simulink model "PEMFC20220411"  (R2021a)
settings: Solver=VariableStepAuto  StartTime=0.0  StopTime=3500  RelTol=1e-3
settings Model: Creator=workstation  LastModifiedBy=workstation

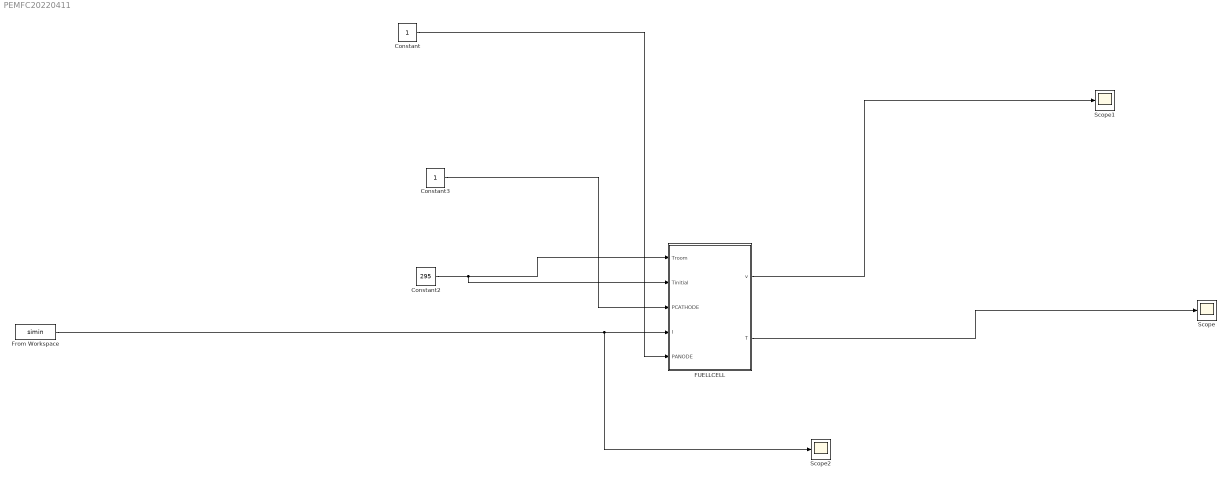
== system PEMFC20220411 ==
  Constant : Constant
  Constant2 : Constant  Value=295
  Constant3 : Constant
  FUELLCELL : Subsystem
  From Workspace : FromWorkspace  VariableName=simin
  Scope : Scope
  Scope1 : Scope
  Scope2 : Scope
  wires:
  Constant2/1 -> FUELLCELL/2(Tinitial), FUELLCELL/1(Troom)
  Constant3/1 -> FUELLCELL/3(PCATHODE)
  From Workspace/1 -> Scope2/1, FUELLCELL/4(I)
  Constant/1 -> FUELLCELL/5(PANODE)
  FUELLCELL/1(v) -> Scope1/1
  FUELLCELL/2(T) -> Scope/1

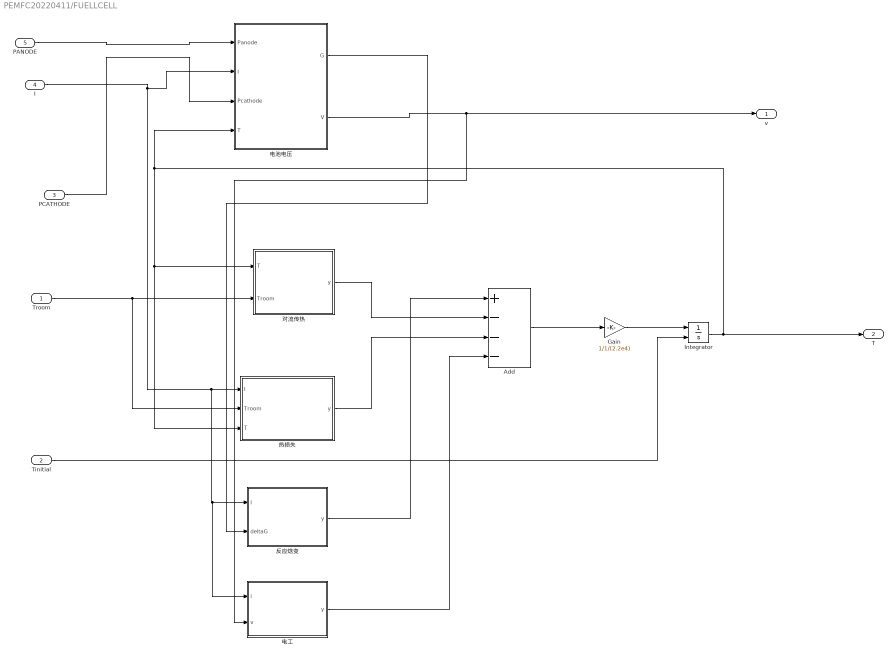
== system PEMFC20220411/FUELLCELL ==
  Troom : Inport
  Tinitial : Inport  Port=2
  PCATHODE : Inport  Port=3
  I : Inport  Port=4
  PANODE : Inport  Port=5
  Add : Sum  Inputs=+---
  Gain : Gain  Gain=1/1/(2.2e4)
  Integrator : Integrator  InitialConditionSource=external
  反应焓变 : MATLAB Function  TreatAsAtomicUnit=on
  对流传热 : MATLAB Function  TreatAsAtomicUnit=on
  热损失 : MATLAB Function  TreatAsAtomicUnit=on
  电工 : MATLAB Function  TreatAsAtomicUnit=on
  电池电压 : Subsystem
  v : Outport
  T : Outport  Port=2
  wires:
  电池电压/2(V) -> v/1, 电工/2(v)
  Integrator/1 -> T/1, 电池电压/4(T), 热损失/3(T), 对流传热/1(T)
  对流传热/1(y) -> Add/2
  Troom/1 -> 热损失/2(Troom), 对流传热/2(Troom)
  Gain/1 -> Integrator/1
  Tinitial/1 -> Integrator/2
  PANODE/1 -> 电池电压/1(Panode)
  热损失/1(y) -> Add/3
  I/1 -> 电工/1(i), 反应焓变/1(I), 热损失/1(I), 电池电压/2(I)
  电池电压/1(G) -> 反应焓变/2(deltaG)
  反应焓变/1(y) -> Add/1
  Add/1 -> Gain/1
  PCATHODE/1 -> 电池电压/3(Pcathode)
  电工/1(y) -> Add/4

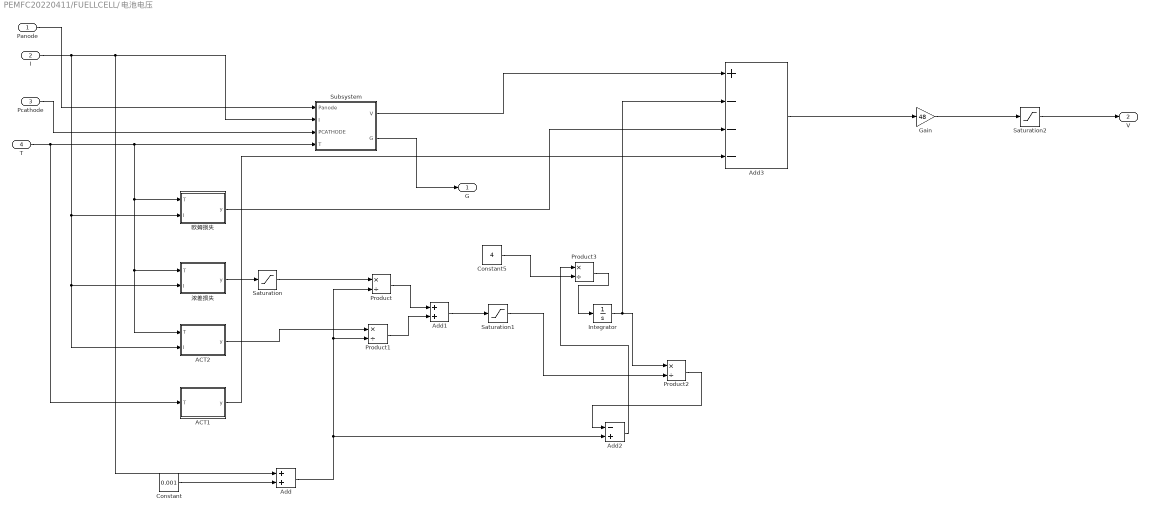
== system PEMFC20220411/FUELLCELL/电池电压 ==
  Panode : Inport
  I : Inport  Port=2
  Pcathode : Inport  Port=3
  T : Inport  Port=4
  ACT1 : MATLAB Function  TreatAsAtomicUnit=on
  ACT2 : MATLAB Function  TreatAsAtomicUnit=on
  Add : Sum
  Add1 : Sum
  Add2 : Sum  Inputs=-+
  Add3 : Sum  Inputs=+---
  Constant : Constant  Value=0.001
  Constant5 : Constant  Value=4
  Gain : Gain  Gain=48
  Integrator : Integrator
  Product{,1..3} (4 alike) : Product  Inputs=*/
  Saturation : Saturate  UpperLimit=1  LowerLimit=0
  Saturation1 : Saturate  UpperLimit=10  LowerLimit=0.00001
  Saturation2 : Saturate  UpperLimit=58  LowerLimit=0
  Subsystem : Subsystem
  欧姆损失 : MATLAB Function  TreatAsAtomicUnit=on
  浓差损失 : MATLAB Function  TreatAsAtomicUnit=on
  G : Outport
  V : Outport  Port=2
  wires:
  Add2/1 -> Product3/1
  Pcathode/1 -> Subsystem/3(PCATHODE)
  Subsystem/1(V) -> Add3/1
  ACT1/1(y) -> Add3/4
  I/1 -> 欧姆损失/2(I), ACT2/2(I), 浓差损失/2(I), Add/1, Subsystem/2(I)
  欧姆损失/1(y) -> Add3/3
  Product1/1 -> Add1/2
  T/1 -> ACT1/1(T), 欧姆损失/1(T), ACT2/1(T), 浓差损失/1(T), Subsystem/4(T)
  Gain/1 -> Saturation2/1
  Add/1 -> Add2/2, Product1/2, Product/2
  Integrator/1 -> Product2/1, Add3/2
  Add1/1 -> Saturation1/1
  Saturation1/1 -> Product2/2
  Product2/1 -> Add2/1
  Product/1 -> Add1/1
  Subsystem/2(G) -> G/1
  浓差损失/1(y) -> Saturation/1
  Add3/1 -> Gain/1
  Panode/1 -> Subsystem/1(Panode)
  Constant/1 -> Add/2
  Constant5/1 -> Product3/2
  Saturation/1 -> Product/1
  Product3/1 -> Integrator/1
  ACT2/1(y) -> Product1/1
  Saturation2/1 -> V/1

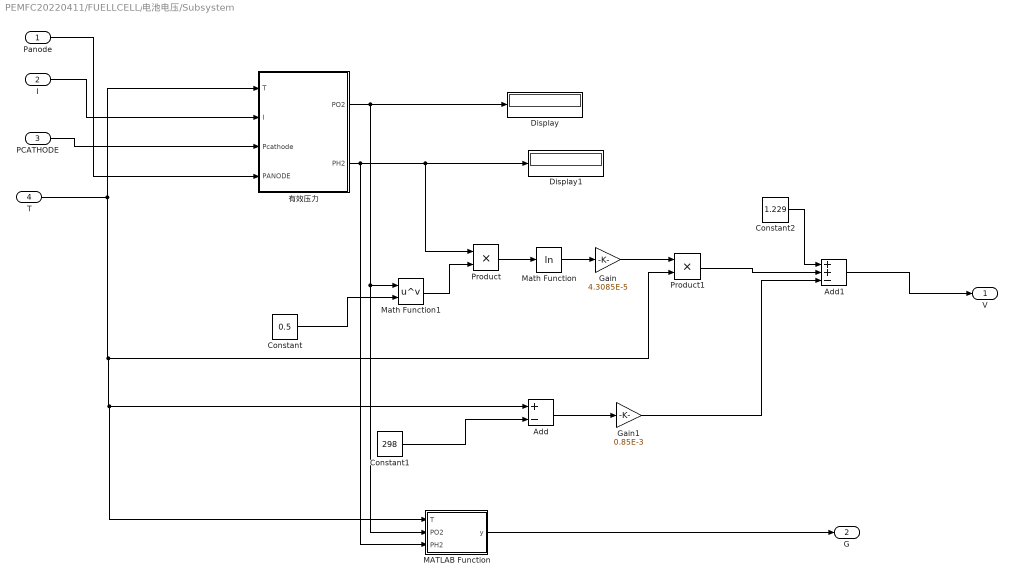
== system PEMFC20220411/FUELLCELL/电池电压/Subsystem ==
  Panode : Inport
  I : Inport  Port=2
  PCATHODE : Inport  Port=3
  T : Inport  Port=4
  Add : Sum  Inputs=+-
  Add1 : Sum  Inputs=++-
  Constant : Constant  Value=0.5
  Constant1 : Constant  Value=298
  Constant2 : Constant  Value=1.229
  Display : Display
  Display1 : Display
  Gain : Gain  Gain=4.3085E-5
  Gain1 : Gain  Gain=0.85E-3
  MATLAB Function : MATLAB Function  TreatAsAtomicUnit=on
  Math Function : Math  Operator=log  SaturateOnIntegerOverflow=on
  Math Function1 : Math  Operator=pow  SaturateOnIntegerOverflow=on
  Product : Product
  Product1 : Product
  有效压力 : Subsystem
  V : Outport
  G : Outport  Port=2
  wires:
  有效压力/1(PO2) -> MATLAB Function/2(PO2), Math Function1/1, Display/1
  I/1 -> 有效压力/2(I)
  有效压力/2(PH2) -> MATLAB Function/3(PH2), Product/1, Display1/1
  T/1 -> MATLAB Function/1(T), Add/1, Product1/2, 有效压力/1(T)
  Add1/1 -> V/1
  PCATHODE/1 -> 有效压力/3(Pcathode)
  Constant1/1 -> Add/2
  Add/1 -> Gain1/1
  Gain1/1 -> Add1/3
  MATLAB Function/1(y) -> G/1
  Constant2/1 -> Add1/1
  Gain/1 -> Product1/1
  Product/1 -> Math Function/1
  Math Function1/1 -> Product/2
  Product1/1 -> Add1/2
  Constant/1 -> Math Function1/2
  Math Function/1 -> Gain/1
  Panode/1 -> 有效压力/4(PANODE)

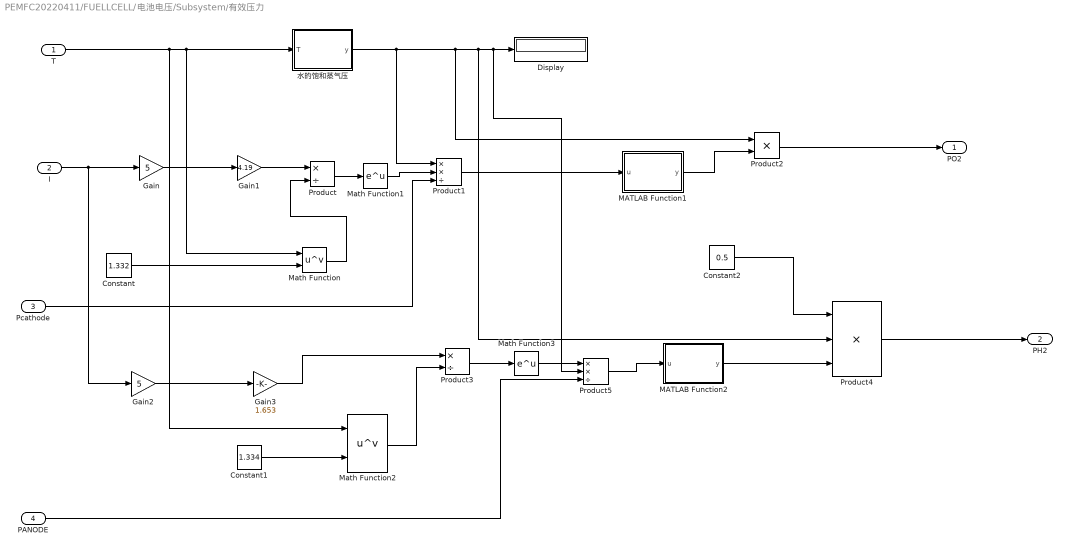
== system PEMFC20220411/FUELLCELL/电池电压/Subsystem/有效压力 ==
  T : Inport
  I : Inport  Port=2
  Pcathode : Inport  Port=3
  PANODE : Inport  Port=4
  Constant : Constant  Value=1.332
  Constant1 : Constant  Value=1.334
  Constant2 : Constant  Value=0.5
  Display : Display
  Gain : Gain  Gain=5
  Gain1 : Gain  Gain=4.19
  Gain2 : Gain  Gain=5
  Gain3 : Gain  Gain=1.653
  MATLAB Function1 : MATLAB Function  TreatAsAtomicUnit=on
  MATLAB Function2 : MATLAB Function  TreatAsAtomicUnit=on
  Math Function : Math  Operator=pow  SaturateOnIntegerOverflow=on
  Math Function1 : Math  SaturateOnIntegerOverflow=on
  Math Function2 : Math  Operator=pow  SaturateOnIntegerOverflow=on
  Math Function3 : Math  SaturateOnIntegerOverflow=on
  Product : Product  Inputs=*/
  Product1 : Product  Inputs=**/
  Product2 : Product
  Product3 : Product  Inputs=*/
  Product4 : Product  Inputs=***
  Product5 : Product  Inputs=**/
  水的饱和蒸气压 : MATLAB Function  TreatAsAtomicUnit=on
  PO2 : Outport
  PH2 : Outport  Port=2
  wires:
  T/1 -> Math Function2/1, Math Function/1, 水的饱和蒸气压/1(T)
  Math Function/1 -> Product/2
  Gain1/1 -> Product/1
  水的饱和蒸气压/1(y) -> Product1/1, Product2/1, Product4/2, Product5/2, Display/1
  Math Function1/1 -> Product1/2
  Constant/1 -> Math Function/2
  Product1/1 -> MATLAB Function1/1(u)
  I/1 -> Gain2/1, Gain/1
  Product2/1 -> PO2/1
  PANODE/1 -> Product5/3
  Constant2/1 -> Product4/1
  Pcathode/1 -> Product1/3
  Gain/1 -> Gain1/1
  Product5/1 -> MATLAB Function2/1(u)
  MATLAB Function2/1(y) -> Product4/3
  Gain3/1 -> Product3/1
  Math Function3/1 -> Product5/1
  Product4/1 -> PH2/1
  MATLAB Function1/1(y) -> Product2/2
  Math Function2/1 -> Product3/2
  Constant1/1 -> Math Function2/2
  Gain2/1 -> Gain3/1
  Product3/1 -> Math Function3/1
  Product/1 -> Math Function1/1

== matlab function PEMFC20220411/FUELLCELL/电池电压/Subsystem/有效压力/水的饱和蒸气压 ==
  data: T input; y output
function y = fcn(T)
U =(-40529.4522405347 + 401.94033912153 * T - 1.33430273535993 * (T ^ 2) + 0.00148378443819808 * (  T ^3)) / 760;
y = U;

== matlab function PEMFC20220411/FUELLCELL/电池电压/Subsystem/有效压力/MATLAB Function2 ==
  data: u input; y output
function y = fcn(u)
k = abs(1/u-1);
y = k;

== matlab function PEMFC20220411/FUELLCELL/电池电压/Subsystem/MATLAB Function ==
  data: T input; y output; PO2 input; PH2 input
function y = fcn(T,PO2, PH2)
DELTAG = 237200 - ((T - 298.15) * 0.163) + (8.31 * (log(PO2^(0.5) * PH2)) * T)
y = DELTAG;

== matlab function PEMFC20220411/FUELLCELL/电池电压/欧姆损失 ==
  data: T input; y output; I input
function y = fcn(T,I)
Ohmic = ((-0.0158 + (3.8e-5) * T) - (3.0e-5 * I)) * I * (-1.3);

y = Ohmic;

== matlab function PEMFC20220411/FUELLCELL/电池电压/浓差损失 ==
  data: T input; y output; I input
function y = fcn(T,I)
con = -2.6 * ((T * 4.3085e-5) * log((abs(1 - I / 25)) + 1.0e-100));
y = con;

== matlab function PEMFC20220411/FUELLCELL/电池电压/ACT2 ==
  data: T input; y output; I input
function y = fcn(T,I)
act2 = T * ((1.87e-4 * log(I + 1)) * 0.40) * 1.3;
y = act2;

== matlab function PEMFC20220411/FUELLCELL/电池电压/ACT1 ==
  data: T input; y output
function y = fcn(T)
act1 = (0.9514 * 1.0284 - 2.2e-3 * T) * 1.3;
y = act1;

== matlab function PEMFC20220411/FUELLCELL/对流传热 ==
  data: T input; y output; Troom input
function y = fcn(T,Troom)
h = 24*3.2e-2*(T-Troom);
y = h;

== matlab function PEMFC20220411/FUELLCELL/热损失 ==
  data: I input; y output; Troom input; T input
function y = fcn(I,Troom,T)
T1 = I * 1 / (2.0 * 96487.0) * 28.68 * (2 * Troom - T);
T2 = I * 1 / (4.0 * 96487.0) * 29.39 * (2 * Troom - T);
T3 = I * 1 / (2.0 * 96487.0) * 75.4 * (T - Troom);
T4 = I *1.0 / (2.0 * 96487.0) * 40644;
T5 = (T1 + T2 + T4 + T3)*48;
y = T5;

== matlab function PEMFC20220411/FUELLCELL/反应焓变 ==
  data: I input; y output; deltaG input
function y = fcn(I,deltaG)
u = I * 1 / (2.0 * 96487.0) * deltaG * 48;
y = u;

== matlab function PEMFC20220411/FUELLCELL/电池电压/Subsystem/有效压力/MATLAB Function1 ==
  data: u input; y output
function y = fcn(u)
k = abs(1/u-1);
y = k;

== matlab function PEMFC20220411/FUELLCELL/电工 ==
  data: i input; y output; v input
function y = fcn(i,v)
u=i*v;
y = u;
